simulink model "verify_PipeStratEnhanced_mdl"  (R2018b)
settings: Solver=VariableStepAuto  StartTime=0.0  StopTime=5*3600  MaxStep=900  RelTol=1e-3  EnableMultiTasking=on
undefined symbols (not defined in the file or in its folder): hgt
libraries: carnot x24, simulink x12
settings Model: Creator=drhf  LastModifiedBy=drhf
settings SolverCC: ZeroCrossAlgorithm=Adaptive
settings DataIOCC: SaveFormat=Array  SignalLoggingSaveFormat=ModelDataLogs
settings OptimizationCC: ExpressionDepthLimit=2147483647  LifeSpan=inf
settings DebuggingCC: UnderspecifiedInitializationDetection=Classic  MergeDetectMultiDrivingBlocksExec=none  MaskedZcDiagnostic=none  IgnoredZcDiagnostic=none  SolverPrmCheckMsg=warning  FcnCallInpInsideContextMsg=warning  StateNameClashWarn=warning  SFUnexpectedBacktrackingDiag=warning  SFNoUnconditionalDefaultTransitionDiag=warning  SFExecutionAtInitializationDiag=none
settings HardwareCC: ProdBitPerPointer=32  ProdBitPerSizeT=32  ProdBitPerPtrDiffT=32  ProdLargestAtomicFloat=None  ProdIntDivRoundTo=Undefined  ProdEndianess=Unspecified  ProdWordSize=32  ProdHWDeviceType=32-bit Generic
settings ModelReferenceCC: PropagateSignalLabelsOutOfModel=off
settings SFSimCC: SimUseLocalCustomCode=off
settings RTWCC: RTWUseLocalCustomCode=off
settings CodeAppCC: StateflowObjectComments=on
settings GRTTargetCC: TargetLangStandard=C89/C90 (ANSI)  GeneratePreprocessorConditionals=Disable all  CombineOutputUpdateFcns=off  GRTInterface=on
settings ConfigComp: CovMetricSettings=dw  CovHtmlReporting=on  CovSaveCumulativeToWorkspaceVar=on  CovSaveSingleToWorkspaceVar=on  CovExternalEMLEnable=off

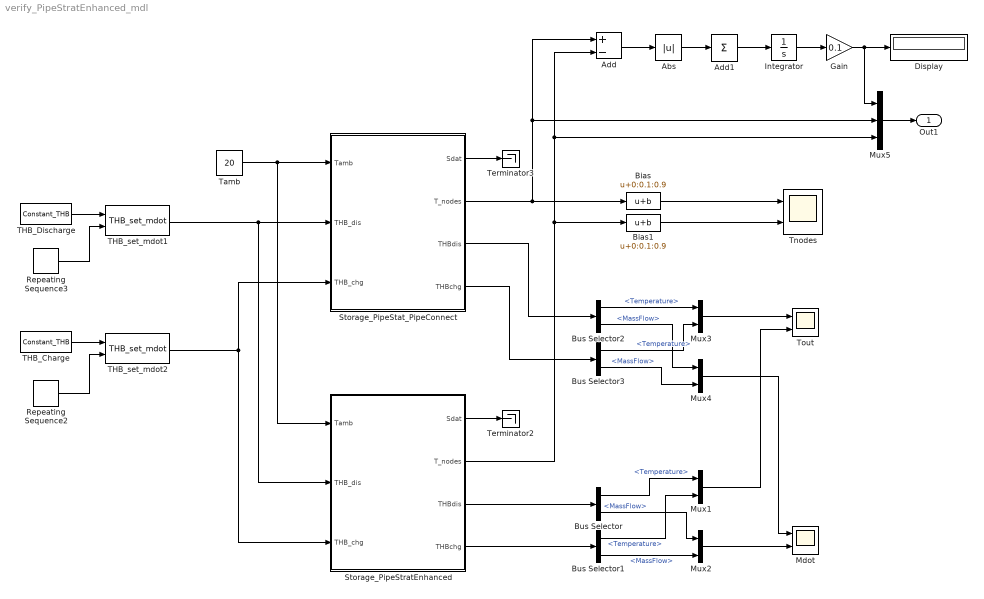
== system verify_PipeStratEnhanced_mdl ==
  Abs : Abs
  Add : Sum  Inputs=+-
  Add1 : Sum  Inputs=1
  Bias : Bias  Bias=0:0.1:0.9
  Bias1 : Bias  Bias=0:0.1:0.9
  Bus Selector{,1..3} (4 alike) : BusSelector  OutputSignals=Temperature,MassFlow
  Display : Display
  Gain : Gain  Gain=0.1
  Integrator : Integrator
  Mdot : Scope  NumInputPorts=2
  Mux{1..4} (4 alike) : Mux  Inputs=2
  Mux5 : Mux  Inputs=3
  Repeating Sequence2 : simulink/Sources/Repeating Sequence  rep_seq_t=[0 0.99 1 1.99 2 2.99 3 3.99 4 5]*3600  rep_seq_y=[0.1 0.1 0 0 1 1 0 0 1 1]*360/3600
  Repeating Sequence3 : simulink/Sources/Repeating Sequence  rep_seq_t=[0 0.99 1 1.99 2 2.99 3 3.99 4 5]*3600  rep_seq_y=[0 0 0.1 0.1 0 0 1 1 0 0]*360/3600
  Storage_PipeStat_PipeConnect : Subsystem  mask(Multiport Storage){uloss=0, ubot=0, utop=0, cond=0, t0=[10 10 10 10 10 70 70 70 70 70], volume=0.3, dia=0.5, pos=standing cylinder, nconnect=4, outlet_charge=1, outlet_discharge=0, nodes=100, mpoints=10}
      mask prompts: uloss "Heat loss coefficient cylinder wall in W/(m²K)"; ubot "Heat loss coefficient bottom in W/(m²K)"; utop "Heat loss coefficient top cover in W/(m²K)"; cond "Effective vertical conductivity in W/(m*K)"; t0 "Initial temperature (vector or scalar) in °C"; volume "Volume in m³"; dia "Diameter in m"; pos "Position"; nconnect "Number of connections"; outlet_charge "Stratified charging pipe outlet"; outlet_discharge "Statified discharging pipe outlet"; nodes "Number of nodes"; mpoints "Number of measurement points"
      mask help:
      | The volmue of the cylindrical storage is divided in a number "nodes" of horizontal slices (1xN-node model). For each node the energy balance equation is solved.
      | Look under mask to set the ports types and properties.
      mask init:
      | [standing, dh, height, mpts, tini] ...
      |     = CarnotCallbacks_StorageTypeN(pos, volume, dia, nodes, mpoints, t0);
      mask Help: eval('man(''storage_multiport'')')
      mask TypeOptions pos: lying cylinder | standing cylinder
      mask DialogControl ParameterTabVar0 Prompt: Thermal
      mask DialogControl ParameterTabVar01 Prompt: Geometry
      mask DialogControl ParameterTabVar012 Prompt: Calculation
      mask Display: plot(10,20,80,100,[36,36,40,50,54,54,50,40,36],[90,50,45,45,50,90,93,93,90],[36,51,44,51,36],[50,50,55,60,60])
  Storage_PipeStratEnhanced : Subsystem  mask(Multiport Storage){uloss=0, ubot=0, utop=0, cond=0, t0=[10 10 10 10 10 70 70 70 70 70], volume=0.3, dia=0.5, pos=standing cylinder, nconnect=2, outlet_charge=1, outlet_discharge=0, nodes=100, mpoints=10}
      mask prompts: uloss "Heat loss coefficient cylinder wall in W/(m²K)"; ubot "Heat loss coefficient bottom in W/(m²K)"; utop "Heat loss coefficient top cover in W/(m²K)"; cond "Effective vertical conductivity in W/(m*K)"; t0 "Initial temperature (vector or scalar) in °C"; volume "Volume in m³"; dia "Diameter in m"; pos "Position"; nconnect "Number of connections"; outlet_charge "Stratified charging pipe outlet"; outlet_discharge "Statified discharging pipe outlet"; nodes "Number of nodes"; mpoints "Number of measurement points"
      mask help:
      | The volmue of the cylindrical storage is divided in a number "nodes" of horizontal slices (1xN-node model). For each node the energy balance equation is solved.
      | Look under mask to set the ports types and properties.
      mask init:
      | [standing, dh, height, mpts, tini] ...
      |     = CarnotCallbacks_StorageTypeN(pos, volume, dia, nodes, mpoints, t0);
      | height = 1;
      mask Help: eval('man(''storage_multiport'')')
      mask TypeOptions pos: lying cylinder | standing cylinder
      mask DialogControl ParameterTabVar0 Prompt: Thermal
      mask DialogControl ParameterTabVar01 Prompt: Geometry
      mask DialogControl ParameterTabVar012 Prompt: Calculation
      mask Display: plot(10,20,80,100,[36,36,40,50,54,54,50,40,36],[90,50,45,45,50,90,93,93,90],[36,51,44,51,36],[50,50,55,60,60])
  THB_Charge : carnot/Source/Simple/Constant_THB  t=50  mdot=0  p=1e5  mID=No Pressure Drop  fluid=Water  mix=0  mix2=0  mix3=0  dia=0.02  hgt=0
      settings: SourceProductName=Carnot
  THB_Discharge : carnot/Source/Simple/Constant_THB  t=20  mdot=0  p=1e5  mID=No Pressure Drop  fluid=Water  mix=0  mix2=0  mix3=0  dia=0.02  hgt=0
      settings: SourceProductName=Carnot
  THB_set_mdot1 : carnot/Source/Simple/THB_set_mdot
      settings: SourceProductName=Carnot
  THB_set_mdot2 : carnot/Source/Simple/THB_set_mdot
      settings: SourceProductName=Carnot
  Tamb : Constant  Value=20
  Terminator2 : Terminator
  Terminator3 : Terminator
  Tnodes : Scope  NumInputPorts=2
  Tout : Scope  NumInputPorts=2
  Out1 : Outport
  wires:
  Tamb/1 -> Storage_PipeStat_PipeConnect/1(Tamb), Storage_PipeStratEnhanced/1(Tamb)
  Storage_PipeStat_PipeConnect/1(Sdat) -> Terminator3/1
  THB_set_mdot1/1 -> Storage_PipeStratEnhanced/2(THB_dis), Storage_PipeStat_PipeConnect/2(THB_dis)
  THB_set_mdot2/1 -> Storage_PipeStat_PipeConnect/3(THB_chg), Storage_PipeStratEnhanced/3(THB_chg)
  Storage_PipeStratEnhanced/1(Sdat) -> Terminator2/1
  Storage_PipeStratEnhanced/3(THBdis) -> Bus Selector/1
  Storage_PipeStratEnhanced/4(THBchg) -> Bus Selector1/1
  THB_Charge/1 -> THB_set_mdot2/1
  THB_Discharge/1 -> THB_set_mdot1/1
  Repeating Sequence3/1 -> THB_set_mdot1/2
  Repeating Sequence2/1 -> THB_set_mdot2/2
  Bus Selector/1 -> Mux1/1  "<Temperature>"
  Bus Selector1/1 -> Mux1/2  "<Temperature>"
  Bus Selector/2 -> Mux2/1  "<MassFlow>"
  Bus Selector1/2 -> Mux2/2  "<MassFlow>"
  Mux2/1 -> Mdot/2
  Mux3/1 -> Tout/1
  Bus Selector3/2 -> Mux4/2  "<MassFlow>"
  Bus Selector2/2 -> Mux4/1  "<MassFlow>"
  Bus Selector3/1 -> Mux3/2  "<Temperature>"
  Bus Selector2/1 -> Mux3/1  "<Temperature>"
  Storage_PipeStat_PipeConnect/4(THBchg) -> Bus Selector3/1
  Storage_PipeStat_PipeConnect/3(THBdis) -> Bus Selector2/1
  Storage_PipeStat_PipeConnect/2(T_nodes) -> Mux5/2, Add/1, Bias/1
  Storage_PipeStratEnhanced/2(T_nodes) -> Mux5/3, Add/2, Bias1/1
  Mux1/1 -> Tout/2
  Mux4/1 -> Mdot/1
  Add/1 -> Abs/1
  Abs/1 -> Add1/1
  Integrator/1 -> Gain/1
  Bias/1 -> Tnodes/1
  Bias1/1 -> Tnodes/2
  Add1/1 -> Integrator/1
  Gain/1 -> Mux5/1, Display/1
  Mux5/1 -> Out1/1

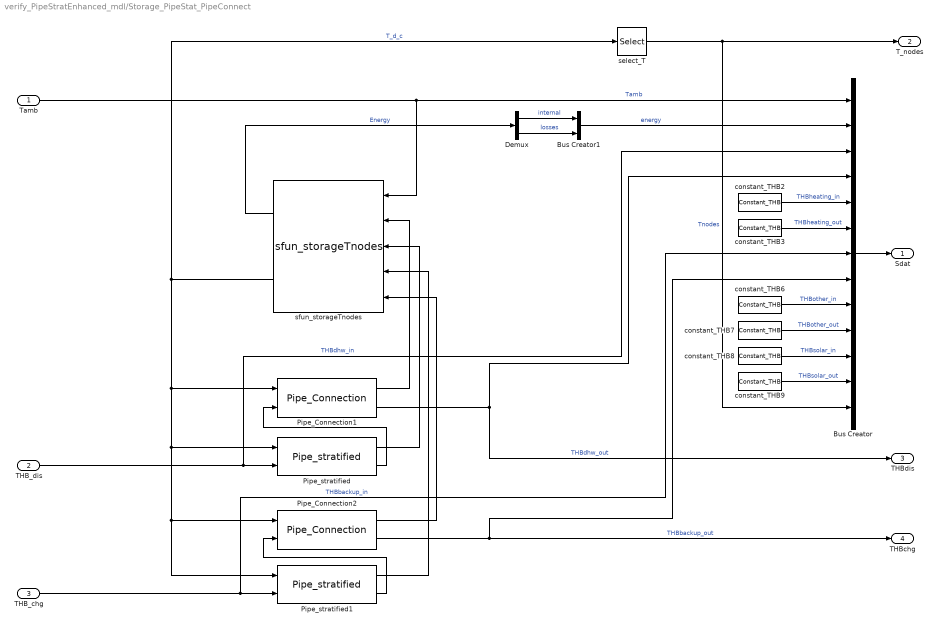
== system verify_PipeStratEnhanced_mdl/Storage_PipeStat_PipeConnect ==
  Tamb : Inport
  THB_dis : Inport  Port=2
  THB_chg : Inport  Port=3
  Bus Creator : BusCreator  Inputs=13
  Bus Creator1 : BusCreator  Inputs=2
  Demux : Demux  Outputs=2
  Pipe_Connection1 : carnot/Storage/Thermal/Storage_Ports/Pipe_Connection  h_in=outlet_discharge  h_out=1  hgt=1  dpipe=0.03  dstg=1  height=1  nodes=nodes
      settings: SourceProductName=Carnot
  Pipe_Connection2 : carnot/Storage/Thermal/Storage_Ports/Pipe_Connection  h_in=outlet_charge  h_out=0  hgt=height  dpipe=0.03  dstg=1  height=-1.5279  nodes=nodes
      settings: SourceProductName=Carnot
  Pipe_stratified : carnot/Storage/Thermal/Storage_Ports/Pipe_stratified  h_in=0  h_out=outlet_discharge  hgt=1  dpipe=0.02  dstg=1  height=0  nodes=nodes
      settings: SourceProductName=Carnot
  Pipe_stratified1 : carnot/Storage/Thermal/Storage_Ports/Pipe_stratified  h_in=1  h_out=outlet_charge  hgt=1  dpipe=0.02  dstg=1  height=0  nodes=nodes
      settings: SourceProductName=Carnot
  constant_THB{2..3,6..9} (6 alike) : carnot/Source/Simple/Constant_THB  t=20  mdot=0  p=1e5  mID=No Pressure Drop  fluid=Water  mix=0  mix2=0  mix3=0  dia=0.02  hgt=0
      settings: SourceProductName=Carnot
  select_T : Selector  InputPortWidth=nodes  IndexOptions=Index vector (dialog)  Indices=mpts  OutputSizes=1
  sfun_storageTnodes : carnot/Basic/Thermal_Models/sfun_storageTnodes  uloss=uloss  ubot=ubot  utop=utop  cond=cond  volume=volume  dia=dia  standing=standing cylinder  tini=tini  nodes=nodes  nconnect=nconnect  elimthermocline=2  condinvtc=1e5
      settings: SourceProductName=Carnot
  Sdat : Outport
  T_nodes : Outport  Port=2
  THBdis : Outport  Port=3
  THBchg : Outport  Port=4
  wires:
  Tamb/1 -> sfun_storageTnodes/1, Bus Creator/1  "Tamb"
  THB_dis/1 -> Bus Creator/3, Pipe_stratified/2  "THBdhw_in"
  Pipe_Connection1/2 -> THBdis/1, Bus Creator/4  "THBdhw_out"
  Pipe_Connection1/1 -> sfun_storageTnodes/2
  select_T/1 -> Bus Creator/13, T_nodes/1  "Tnodes"
  sfun_storageTnodes/1 -> Demux/1  "Energy"
  sfun_storageTnodes/2 -> Pipe_stratified/1, Pipe_stratified1/1, Pipe_Connection2/1, Pipe_Connection1/1, select_T/1  "T_d_c"
  Bus Creator/1 -> Sdat/1
  constant_THB9/1 -> Bus Creator/12  "THBsolar_out"
  constant_THB8/1 -> Bus Creator/11  "THBsolar_in"
  constant_THB7/1 -> Bus Creator/10  "THBother_out"
  constant_THB6/1 -> Bus Creator/9  "THBother_in"
  constant_THB2/1 -> Bus Creator/5  "THBheating_in"
  constant_THB3/1 -> Bus Creator/6  "THBheating_out"
  THB_chg/1 -> Bus Creator/7, Pipe_stratified1/2  "THBbackup_in"
  Pipe_Connection2/2 -> Bus Creator/8, THBchg/1  "THBbackup_out"
  Pipe_Connection2/1 -> sfun_storageTnodes/5
  Demux/1 -> Bus Creator1/1  "internal"
  Demux/2 -> Bus Creator1/2  "losses"
  Bus Creator1/1 -> Bus Creator/2  "energy"
  Pipe_stratified/1 -> sfun_storageTnodes/3
  Pipe_stratified/2 -> Pipe_Connection1/2
  Pipe_stratified1/1 -> sfun_storageTnodes/4
  Pipe_stratified1/2 -> Pipe_Connection2/2

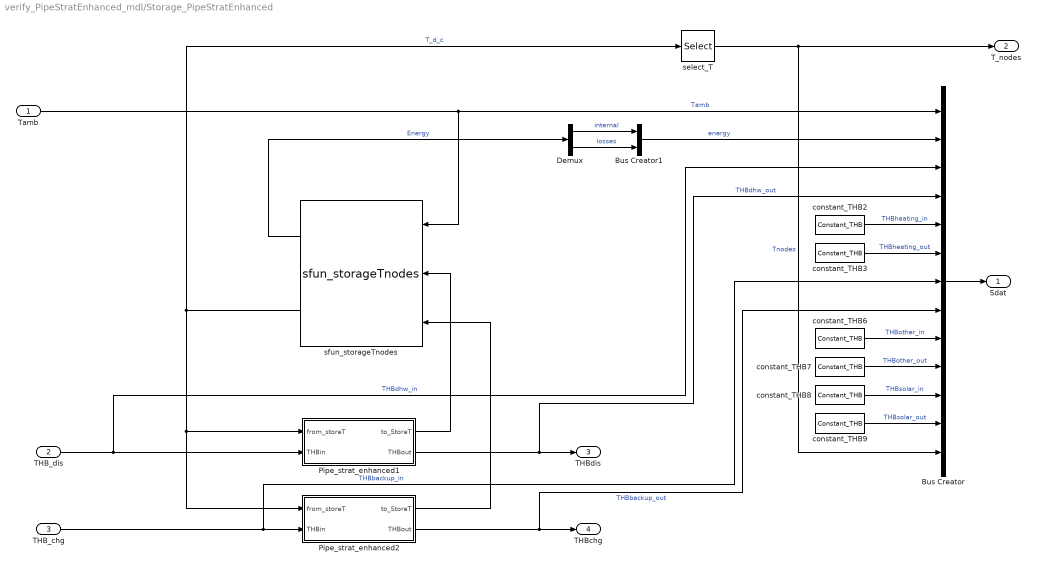
== system verify_PipeStratEnhanced_mdl/Storage_PipeStratEnhanced ==
  Tamb : Inport
  THB_dis : Inport  Port=2
  THB_chg : Inport  Port=3
  Bus Creator : BusCreator  Inputs=13
  Bus Creator1 : BusCreator  Inputs=2
  Demux : Demux  Outputs=2
  Pipe_strat_enhanced1 : Subsystem  mask(pipe connection to storage){h_in=0, h_strat=outlet_discharge, h_out=1, hgt=hgt, dia=0.02, height=1, nodes=nodes}
      mask prompts: h_in "relative height of the starting point of the stratification device"; h_strat "relative height of the end point of the stratification device"; h_out "relative height of outlet"; hgt "Height of storage in m"; dia "Diameter of pipe in m"; height "Height difference inlet-outlet"; nodes "Number of nodes (DO NOT CHANGE)"
      mask help:
      | The block transforms the incoming THV vector to a vector which the storage interprets as a flow into the storage fluid.
      | Give inlet- and outlet-height as a relative position from 0 (= bottom) to 1 (= top).
      mask init:
      | in = zeros(nodes,1);    % vector of length nodes
      | up = in;                % vector of length nodes
      | down = in;              % vector of length nodes
      | 
      | h_in = max(0,min(h_in,1));     % no nodes below 0 and above 1
      | h_out = max(0,min(h_out,1));   % no nodes below 0 and above 1
      | h_strat = max(0,min(h_strat,1));   % no nodes below 0 and above 1
      | %set_param(gcb,'height',num2str((h_out-h_in)*hgt));
      | 
      | inlet = max(ceil(h_in*nodes),1);    % inlet position
      | outlet = max(ceil(h_out*nodes),1);  % outlet position
      | strat = max(ceil(h_strat*nodes),1);  % startification position
      | hgt = (h_out-h_in)*hgt;
      | in(inlet)=1;
      | n_concerned = inlet;
      | 
      | idx_in_out = inlet:outlet;
      | if (inlet < outlet && strat < outlet && inlet < strat)      % if outlet above inlet and stratification and inlet below stratification
      |     up(inlet:outlet-1)=1;       % upwards
      |     n_concerned = inlet:strat;
      | end
      | 
      | if (inlet < outlet && strat < outlet && inlet > strat) % if outlet above inlet and stratification and inlet above stratification
      |     up(strat:outlet-1)=1;       % upwards
      |     n_concerned = strat:inlet;
      | end
      | 
      | if (inlet < outlet && strat > outlet)                  % if outlet above inlet and below stratification
      |     up(inlet:outlet-1)=1;       % upwards and
      |     down(outlet:strat-1)=1;     % downwards
      |     n_concerned = inlet:strat;
      | end
      | 
      | if (inlet > outlet && strat < outlet)                  % if outlet below inlet and above stratification
      |     up(strat:outlet-1)=1;       % upwars and
      |     down(outlet:inlet-1)=1;     % downwards
      |     n_concerned = strat:inlet;
      |     idx_in_out = outlet:inlet;
      | end
      | 
      | % if (inlet > outlet && inlet > strat)                    % if inlet above outlet and above stratification
      | if (inlet > outlet && inlet >= strat)                    % if inlet above outlet and above stratification
      |     down(outlet:inlet-1)=1;     % downwards
      |     n_concerned = strat:inlet;                              % if inlet above outlet and below stratification
      |     idx_in_out = outlet:inlet;
      | end
      | 
      | if (inlet > outlet && inlet < strat)
      |     down(outlet:strat-1)=1;     % downwards
      |     n_concerned = inlet:strat;
      |     idx_in_out = outlet:inlet;
      | end
      mask Help: web(fullfile(path_carnot('help'),'StoragePorts_PipeConnections.html'),'-helpbrowser')
      mask TypeOptions dia: Pressure_Drop_StoragePipe/dpipe
      mask TypeOptions height: Pressure_Drop_StoragePipe/hgt
      mask DialogControl ParameterTabVar0 Prompt: Geometry
      mask DialogControl ParameterTabVar02 Prompt: Calculation
      mask Display: disp('Pipe STRAT')
  Pipe_strat_enhanced2 : Subsystem  mask(pipe connection to storage){h_in=1, h_strat=outlet_charge, h_out=0, hgt=hgt, dia=0.02, height=1, nodes=nodes}
      mask prompts: h_in "relative height of the starting point of the stratification device"; h_strat "relative height of the end point of the stratification device"; h_out "relative height of outlet"; hgt "Height of storage in m"; dia "Diameter of pipe in m"; height "Height difference inlet-outlet"; nodes "Number of nodes (DO NOT CHANGE)"
      mask help:
      | The block transforms the incoming THV vector to a vector which the storage interprets as a flow into the storage fluid.
      | Give inlet- and outlet-height as a relative position from 0 (= bottom) to 1 (= top).
      mask init:
      | in = zeros(nodes,1);    % vector of length nodes
      | up = in;                % vector of length nodes
      | down = in;              % vector of length nodes
      | 
      | h_in = max(0,min(h_in,1));     % no nodes below 0 and above 1
      | h_out = max(0,min(h_out,1));   % no nodes below 0 and above 1
      | h_strat = max(0,min(h_strat,1));   % no nodes below 0 and above 1
      | %set_param(gcb,'height',num2str((h_out-h_in)*hgt));
      | 
      | inlet = max(ceil(h_in*nodes),1);    % inlet position
      | outlet = max(ceil(h_out*nodes),1);  % outlet position
      | strat = max(ceil(h_strat*nodes),1);  % startification position
      | hgt = (h_out-h_in)*hgt;
      | in(inlet)=1;
      | n_concerned = inlet;
      | 
      | idx_in_out = inlet:outlet;
      | if (inlet < outlet && strat < outlet && inlet < strat)      % if outlet above inlet and stratification and inlet below stratification
      |     up(inlet:outlet-1)=1;       % upwards
      |     n_concerned = inlet:strat;
      | end
      | 
      | if (inlet < outlet && strat < outlet && inlet > strat) % if outlet above inlet and stratification and inlet above stratification
      |     up(strat:outlet-1)=1;       % upwards
      |     n_concerned = strat:inlet;
      | end
      | 
      | if (inlet < outlet && strat > outlet)                  % if outlet above inlet and below stratification
      |     up(inlet:outlet-1)=1;       % upwards and
      |     down(outlet:strat-1)=1;     % downwards
      |     n_concerned = inlet:strat;
      | end
      | 
      | if (inlet > outlet && strat < outlet)                  % if outlet below inlet and above stratification
      |     up(strat:outlet-1)=1;       % upwars and
      |     down(outlet:inlet-1)=1;     % downwards
      |     n_concerned = strat:inlet;
      |     idx_in_out = outlet:inlet;
      | end
      | 
      | % if (inlet > outlet && inlet > strat)                    % if inlet above outlet and above stratification
      | if (inlet > outlet && inlet >= strat)                    % if inlet above outlet and above stratification
      |     down(outlet:inlet-1)=1;     % downwards
      |     n_concerned = strat:inlet;                              % if inlet above outlet and below stratification
      |     idx_in_out = outlet:inlet;
      | end
      | 
      | if (inlet > outlet && inlet < strat)
      |     down(outlet:strat-1)=1;     % downwards
      |     n_concerned = inlet:strat;
      |     idx_in_out = outlet:inlet;
      | end
      mask Help: web(fullfile(path_carnot('help'),'StoragePorts_PipeConnections.html'),'-helpbrowser')
      mask TypeOptions dia: Pressure_Drop_StoragePipe/dpipe
      mask TypeOptions height: Pressure_Drop_StoragePipe/hgt
      mask DialogControl ParameterTabVar0 Prompt: Geometry
      mask DialogControl ParameterTabVar02 Prompt: Calculation
      mask Display: disp('Pipe STRAT')
  constant_THB{2..3,6..9} (6 alike) : carnot/Source/Simple/Constant_THB  t=20  mdot=0  p=1e5  mID=No Pressure Drop  fluid=Water  mix=0  mix2=0  mix3=0  dia=0.02  hgt=0
      settings: SourceProductName=Carnot
  select_T : Selector  InputPortWidth=nodes  IndexOptions=Index vector (dialog)  Indices=mpts  OutputSizes=1
  sfun_storageTnodes : carnot/Basic/Thermal_Models/sfun_storageTnodes  uloss=uloss  ubot=ubot  utop=utop  cond=cond  volume=volume  dia=dia  standing=standing cylinder  tini=tini  nodes=nodes  nconnect=nconnect  elimthermocline=2  condinvtc=1e5
      settings: SourceProductName=Carnot
  Sdat : Outport
  T_nodes : Outport  Port=2
  THBdis : Outport  Port=3
  THBchg : Outport  Port=4
  wires:
  Bus Creator1/1 -> Bus Creator/2  "energy"
  Demux/2 -> Bus Creator1/2  "losses"
  Demux/1 -> Bus Creator1/1  "internal"
  Pipe_strat_enhanced2/1(to_StoreT) -> sfun_storageTnodes/3
  Pipe_strat_enhanced2/2(THBout) -> Bus Creator/8, THBchg/1  "THBbackup_out"
  THB_chg/1 -> Bus Creator/7, Pipe_strat_enhanced2/2(THBin)  "THBbackup_in"
  constant_THB3/1 -> Bus Creator/6  "THBheating_out"
  constant_THB2/1 -> Bus Creator/5  "THBheating_in"
  constant_THB6/1 -> Bus Creator/9  "THBother_in"
  constant_THB7/1 -> Bus Creator/10  "THBother_out"
  constant_THB8/1 -> Bus Creator/11  "THBsolar_in"
  constant_THB9/1 -> Bus Creator/12  "THBsolar_out"
  Bus Creator/1 -> Sdat/1
  sfun_storageTnodes/2 -> select_T/1, Pipe_strat_enhanced2/1(from_storeT), Pipe_strat_enhanced1/1(from_storeT)  "T_d_c"
  sfun_storageTnodes/1 -> Demux/1  "Energy"
  select_T/1 -> T_nodes/1, Bus Creator/13  "Tnodes"
  Pipe_strat_enhanced1/1(to_StoreT) -> sfun_storageTnodes/2
  Pipe_strat_enhanced1/2(THBout) -> THBdis/1, Bus Creator/4  "THBdhw_out"
  THB_dis/1 -> Pipe_strat_enhanced1/2(THBin), Bus Creator/3  "THBdhw_in"
  Tamb/1 -> Bus Creator/1, sfun_storageTnodes/1  "Tamb"

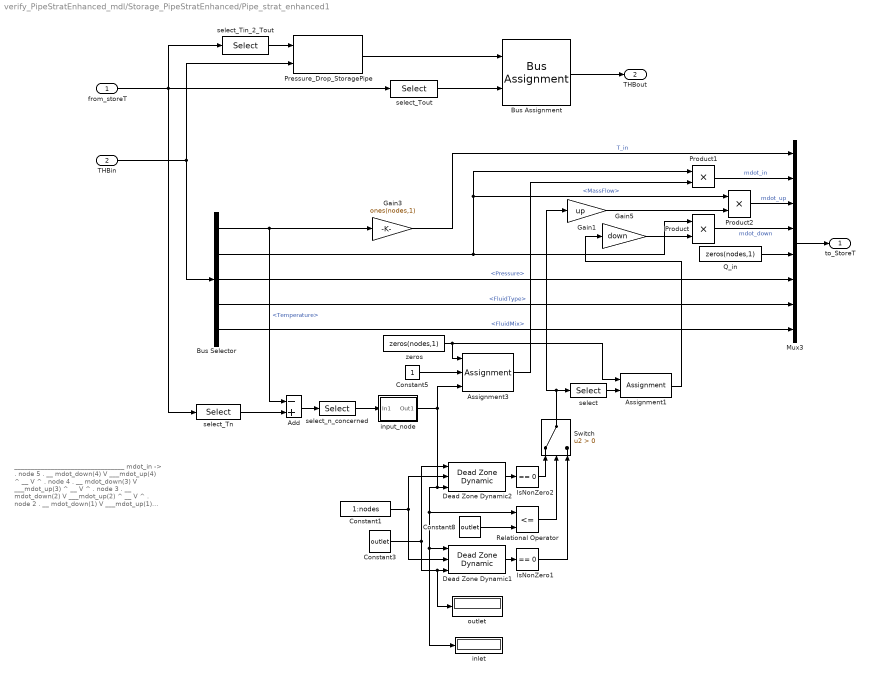
== system verify_PipeStratEnhanced_mdl/Storage_PipeStratEnhanced/Pipe_strat_enhanced1 ==
  note: _________________________________
      | mdot_in ->                                                .
      | node 5                     .
      | __ mdot_down(4) V  ___mdot_up(4) ^ __
      | V                           ^    .
      | node 4                    .
      | __ mdot_down(3) V  ___mdot_up(3) ^ __
      | V                           ^    .
      | node 3                    .
      | __ mdot_down(2) V  ___mdot_up(2) ^ __
      | V                           ^    .
      | node 2                    .
      | __ mdot_down(1) V  ___mdot_up(1) ^ __
      | V                           ^    .
      | node 1                    .
      | _________________________________
  from_storeT : Inport
  THBin : Inport  Port=2
  Add : Sum  Inputs=-+
  Assignment1 : Assignment  DiagnosticForDimensions=Warning  IndexOptions=Index vector (dialog)  Indices=1:nodes-1  OutputSizes=1
  Assignment3 : Assignment  DiagnosticForDimensions=Warning  IndexOptions=Index vector (port)  Indices=1:nodes-1  OutputSizes=1
  Bus Assignment : BusAssignment  AssignedSignals=Temperature
  Bus Selector : BusSelector  OutputSignals=Temperature,MassFlow,Pressure,FluidType,FluidMix
  Constant1 : Constant  Value=1:nodes
  Constant3 : Constant  Value=outlet
  Constant5 : Constant
  Constant8 : Constant  Value=outlet
  Dead Zone Dynamic1 : simulink/Discontinuities/Dead Zone Dynamic
      settings: SourceProductBaseCode=SL
  Dead Zone Dynamic2 : simulink/Discontinuities/Dead Zone Dynamic
      settings: SourceProductBaseCode=SL
  Gain1 : Gain  Gain=up
  Gain3 : Gain  Gain=ones(nodes,1)
  Gain5 : Gain  Gain=down
  IsNonZero1 : simulink/Logic and Bit Operations/Compare To Zero  relop===  OutDataTypeStr=boolean
  IsNonZero2 : simulink/Logic and Bit Operations/Compare To Zero  relop===  OutDataTypeStr=boolean
  Mux3 : Mux  Inputs=8
  Pressure_Drop_StoragePipe : carnot/Basic/Pressure_Drop/Pressure_Drop_StoragePipe  dpipe=dia  dstg=1  hgt=height
      settings: SourceProductName=Carnot
  Product : Product  RndMeth=Zero
  Product1 : Product  RndMeth=Zero
  Product2 : Product  RndMeth=Zero
  Q_in : Constant  Value=zeros(nodes,1)
  Relational Operator : RelationalOperator  Operator=<=  OutDataTypeStr=boolean  RndMeth=Simplest
  Switch : Switch  Criteria=u2 > Threshold
  inlet : Display
  input_node : Subsystem
  outlet : Display
  select : Selector  InputPortWidth=nodes  IndexOptions=Index vector (dialog)  Indices=2:nodes  OutputSizes=1
  select_Tin_2_Tout : Selector  InputPortWidth=nodes  IndexOptions=Index vector (dialog)  Indices=[idx_in_out]  OutputSizes=1
  select_Tn : Selector  InputPortWidth=nodes  IndexOptions=Index vector (dialog)  Indices=[1:nodes]  OutputSizes=1
  select_Tout : Selector  InputPortWidth=nodes  IndexOptions=Index vector (dialog)  Indices=[outlet]  OutputSizes=1
  select_n_concerned : Selector  InputPortWidth=nodes  IndexOptions=Index vector (dialog)  Indices=n_concerned  OutputSizes=1
  zeros : Constant  Value=zeros(nodes,1)
  to_StoreT : Outport
  THBout : Outport  Port=2
  wires:
  zeros/1 -> Assignment3/1, Assignment1/1
  Constant5/1 -> Assignment3/2
  Constant1/1 -> Dead Zone Dynamic2/2, Dead Zone Dynamic1/2
  select/1 -> Assignment1/2
  IsNonZero2/1 -> Switch/1
  Dead Zone Dynamic2/1 -> IsNonZero2/1
  Constant3/1 -> outlet/1, Dead Zone Dynamic1/3, Dead Zone Dynamic2/1
  IsNonZero1/1 -> Switch/3
  input_node/1(Out1) -> Assignment3/3, Dead Zone Dynamic2/3, Relational Operator/1, inlet/1, Dead Zone Dynamic1/1
  Mux3/1 -> to_StoreT/1
  Switch/1 -> select/1, Gain1/1
  select_n_concerned/1 -> input_node/1(In1)
  Assignment1/1 -> Gain5/1
  Relational Operator/1 -> Switch/2
  Constant8/1 -> Relational Operator/2
  Dead Zone Dynamic1/1 -> IsNonZero1/1
  Assignment3/1 -> Product1/2
  Add/1 -> select_n_concerned/1
  Product2/1 -> Mux3/3  "mdot_up"
  select_Tn/1 -> Add/2
  Bus Selector/5 -> Mux3/8  "<FluidMix>"
  Bus Assignment/1 -> THBout/1
  Q_in/1 -> Mux3/5
  Gain3/1 -> Mux3/1  "T_in"
  select_Tout/1 -> Bus Assignment/2
  Bus Selector/1 -> Add/1, Gain3/1  "<Temperature>"
  Bus Selector/2 -> Product1/1, Product2/1, Product/1  "<MassFlow>"
  Bus Selector/3 -> Mux3/6  "<Pressure>"
  Bus Selector/4 -> Mux3/7  "<FluidType>"
  THBin/1 -> Bus Selector/1, Pressure_Drop_StoragePipe/2
  from_storeT/1 -> select_Tout/1, select_Tn/1, select_Tin_2_Tout/1
  Product/1 -> Mux3/4  "mdot_down"
  Gain5/1 -> Product/2
  Product1/1 -> Mux3/2  "mdot_in"
  Pressure_Drop_StoragePipe/1 -> Bus Assignment/1
  select_Tin_2_Tout/1 -> Pressure_Drop_StoragePipe/1
  Gain1/1 -> Product2/2

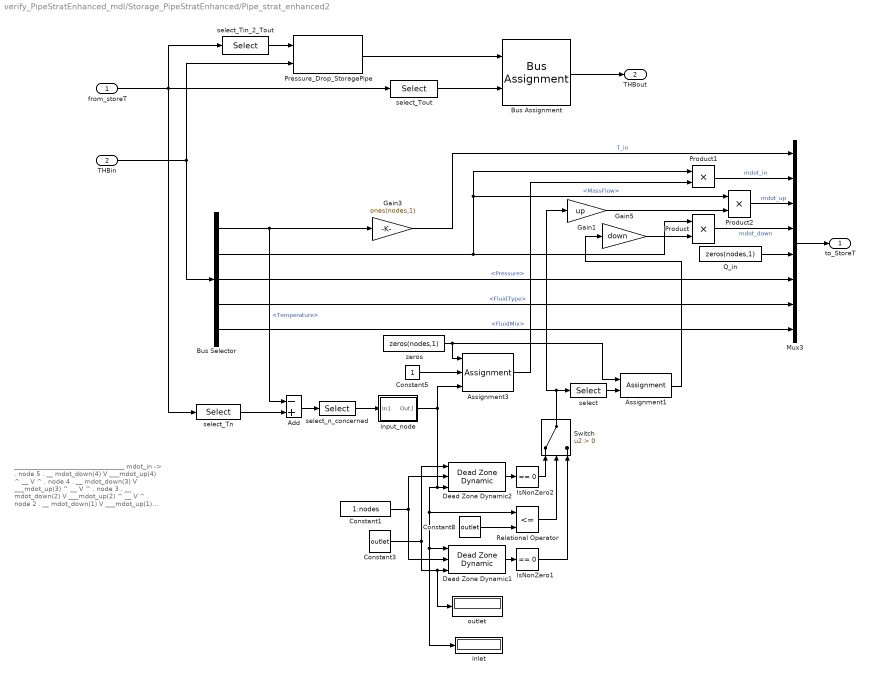
== system verify_PipeStratEnhanced_mdl/Storage_PipeStratEnhanced/Pipe_strat_enhanced2 ==
  note: _________________________________
      | mdot_in ->                                                .
      | node 5                     .
      | __ mdot_down(4) V  ___mdot_up(4) ^ __
      | V                           ^    .
      | node 4                    .
      | __ mdot_down(3) V  ___mdot_up(3) ^ __
      | V                           ^    .
      | node 3                    .
      | __ mdot_down(2) V  ___mdot_up(2) ^ __
      | V                           ^    .
      | node 2                    .
      | __ mdot_down(1) V  ___mdot_up(1) ^ __
      | V                           ^    .
      | node 1                    .
      | _________________________________
  from_storeT : Inport
  THBin : Inport  Port=2
  Add : Sum  Inputs=-+
  Assignment1 : Assignment  DiagnosticForDimensions=Warning  IndexOptions=Index vector (dialog)  Indices=1:nodes-1  OutputSizes=1
  Assignment3 : Assignment  DiagnosticForDimensions=Warning  IndexOptions=Index vector (port)  Indices=1:nodes-1  OutputSizes=1
  Bus Assignment : BusAssignment  AssignedSignals=Temperature
  Bus Selector : BusSelector  OutputSignals=Temperature,MassFlow,Pressure,FluidType,FluidMix
  Constant1 : Constant  Value=1:nodes
  Constant3 : Constant  Value=outlet
  Constant5 : Constant
  Constant8 : Constant  Value=outlet
  Dead Zone Dynamic1 : simulink/Discontinuities/Dead Zone Dynamic
      settings: SourceProductBaseCode=SL
  Dead Zone Dynamic2 : simulink/Discontinuities/Dead Zone Dynamic
      settings: SourceProductBaseCode=SL
  Gain1 : Gain  Gain=up
  Gain3 : Gain  Gain=ones(nodes,1)
  Gain5 : Gain  Gain=down
  IsNonZero1 : simulink/Logic and Bit Operations/Compare To Zero  relop===  OutDataTypeStr=boolean
  IsNonZero2 : simulink/Logic and Bit Operations/Compare To Zero  relop===  OutDataTypeStr=boolean
  Mux3 : Mux  Inputs=8
  Pressure_Drop_StoragePipe : carnot/Basic/Pressure_Drop/Pressure_Drop_StoragePipe  dpipe=dia  dstg=1  hgt=height
      settings: SourceProductName=Carnot
  Product : Product  RndMeth=Zero
  Product1 : Product  RndMeth=Zero
  Product2 : Product  RndMeth=Zero
  Q_in : Constant  Value=zeros(nodes,1)
  Relational Operator : RelationalOperator  Operator=<=  OutDataTypeStr=boolean  RndMeth=Simplest
  Switch : Switch  Criteria=u2 > Threshold
  inlet : Display
  input_node : Subsystem
  outlet : Display
  select : Selector  InputPortWidth=nodes  IndexOptions=Index vector (dialog)  Indices=2:nodes  OutputSizes=1
  select_Tin_2_Tout : Selector  InputPortWidth=nodes  IndexOptions=Index vector (dialog)  Indices=[idx_in_out]  OutputSizes=1
  select_Tn : Selector  InputPortWidth=nodes  IndexOptions=Index vector (dialog)  Indices=[1:nodes]  OutputSizes=1
  select_Tout : Selector  InputPortWidth=nodes  IndexOptions=Index vector (dialog)  Indices=[outlet]  OutputSizes=1
  select_n_concerned : Selector  InputPortWidth=nodes  IndexOptions=Index vector (dialog)  Indices=n_concerned  OutputSizes=1
  zeros : Constant  Value=zeros(nodes,1)
  to_StoreT : Outport
  THBout : Outport  Port=2
  wires:
  Gain1/1 -> Product2/2
  select_Tin_2_Tout/1 -> Pressure_Drop_StoragePipe/1
  Pressure_Drop_StoragePipe/1 -> Bus Assignment/1
  Product1/1 -> Mux3/2  "mdot_in"
  Gain5/1 -> Product/2
  Product/1 -> Mux3/4  "mdot_down"
  from_storeT/1 -> select_Tin_2_Tout/1, select_Tn/1, select_Tout/1
  THBin/1 -> Pressure_Drop_StoragePipe/2, Bus Selector/1
  Bus Selector/4 -> Mux3/7  "<FluidType>"
  Bus Selector/3 -> Mux3/6  "<Pressure>"
  Bus Selector/2 -> Product/1, Product2/1, Product1/1  "<MassFlow>"
  Bus Selector/1 -> Gain3/1, Add/1  "<Temperature>"
  select_Tout/1 -> Bus Assignment/2
  Gain3/1 -> Mux3/1  "T_in"
  Q_in/1 -> Mux3/5
  Bus Assignment/1 -> THBout/1
  Bus Selector/5 -> Mux3/8  "<FluidMix>"
  select_Tn/1 -> Add/2
  Product2/1 -> Mux3/3  "mdot_up"
  Add/1 -> select_n_concerned/1
  Assignment3/1 -> Product1/2
  Dead Zone Dynamic1/1 -> IsNonZero1/1
  Constant8/1 -> Relational Operator/2
  Relational Operator/1 -> Switch/2
  Assignment1/1 -> Gain5/1
  select_n_concerned/1 -> input_node/1(In1)
  Switch/1 -> Gain1/1, select/1
  Mux3/1 -> to_StoreT/1
  input_node/1(Out1) -> Dead Zone Dynamic1/1, inlet/1, Relational Operator/1, Dead Zone Dynamic2/3, Assignment3/3
  IsNonZero1/1 -> Switch/3
  Constant3/1 -> Dead Zone Dynamic2/1, Dead Zone Dynamic1/3, outlet/1
  Dead Zone Dynamic2/1 -> IsNonZero2/1
  IsNonZero2/1 -> Switch/1
  select/1 -> Assignment1/2
  Constant1/1 -> Dead Zone Dynamic1/2, Dead Zone Dynamic2/2
  Constant5/1 -> Assignment3/2
  zeros/1 -> Assignment1/1, Assignment3/1

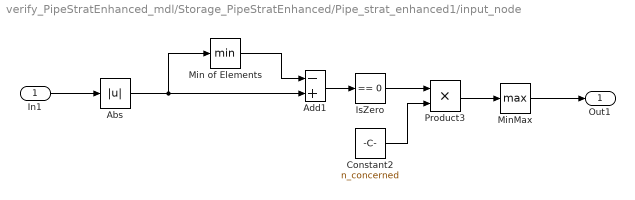
== system verify_PipeStratEnhanced_mdl/Storage_PipeStratEnhanced/Pipe_strat_enhanced1/input_node ==
  In1 : Inport
  Abs : Abs
  Add1 : Sum  Inputs=-+
  Constant2 : Constant  Value=n_concerned
  IsZero : simulink/Logic and Bit Operations/Compare To Zero  relop===  OutDataTypeStr=boolean
  Min of Elements : MinMax
  MinMax : MinMax  Function=max
  Product3 : Product
  Out1 : Outport
  wires:
  Abs/1 -> Add1/2, Min of Elements/1
  MinMax/1 -> Out1/1
  Product3/1 -> MinMax/1
  Add1/1 -> IsZero/1
  Min of Elements/1 -> Add1/1
  IsZero/1 -> Product3/1
  Constant2/1 -> Product3/2
  In1/1 -> Abs/1

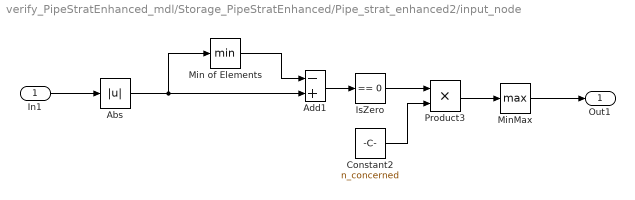
== system verify_PipeStratEnhanced_mdl/Storage_PipeStratEnhanced/Pipe_strat_enhanced2/input_node ==
  In1 : Inport
  Abs : Abs
  Add1 : Sum  Inputs=-+
  Constant2 : Constant  Value=n_concerned
  IsZero : simulink/Logic and Bit Operations/Compare To Zero  relop===  OutDataTypeStr=boolean
  Min of Elements : MinMax
  MinMax : MinMax  Function=max
  Product3 : Product
  Out1 : Outport
  wires:
  In1/1 -> Abs/1
  Constant2/1 -> Product3/2
  IsZero/1 -> Product3/1
  Min of Elements/1 -> Add1/1
  Add1/1 -> IsZero/1
  Product3/1 -> MinMax/1
  MinMax/1 -> Out1/1
  Abs/1 -> Min of Elements/1, Add1/2
